simulink model "ggV_simu"  (R2019a)
settings: Solver=ode1  StartTime=0.0  StopTime=ggV.simu_stopTime  FixedStep=ggV.simu_stepSize  RelTol=1e-3
values from neighbouring files (symbols this model uses):
  init =     [course_data_0_1m.mat]
undefined symbols (not defined in the file or in its folder): ggV_v
settings Model: Creator=Frieder Uerlings  LastModifiedBy=Frieder Uerlings

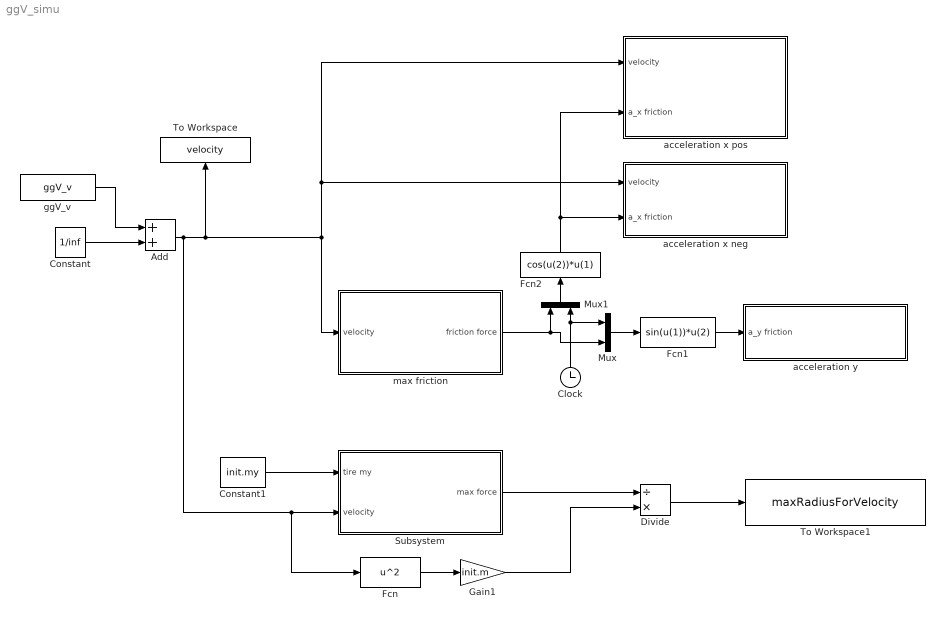
== system ggV_simu ==
  Add : Sum
  Clock : Clock
  Constant : Constant  Value=1/inf
  Constant1 : Constant  Value=init.my
  Divide : Product  Inputs=/*
  Fcn : Fcn  Expr=u^2
  Fcn1 : Fcn  Expr=sin(u(1))*u(2)
  Fcn2 : Fcn  Expr=cos(u(2))*u(1)
  Gain1 : Gain  Gain=init.m
  Mux : Mux  Inputs=2
  Mux1 : Mux  Inputs=2
  Subsystem : Subsystem
  To Workspace : ToWorkspace  VariableName=velocity  SampleTime=-1
  To Workspace1 : ToWorkspace  VariableName=maxRadiusForVelocity  SampleTime=-1
  acceleration x neg : Subsystem
  acceleration x pos : Subsystem
  acceleration y : Subsystem
  "ggV_v " : Constant  Value=ggV_v
  max friction : Subsystem
  wires:
  max friction/1(friction force) -> Mux1/1, Mux/2
  Fcn1/1 -> acceleration y/1(a_y friction)
  Fcn2/1 -> acceleration x pos/2(a_x friction), acceleration x neg/2(a_x friction)
  Add/1 -> Fcn/1, Subsystem/2(velocity), max friction/1(velocity), acceleration x neg/1(velocity), acceleration x pos/1(velocity), To Workspace/1
  Constant/1 -> Add/2
  "ggV_v "/1 -> Add/1
  Mux/1 -> Fcn1/1
  Mux1/1 -> Fcn2/1
  Clock/1 -> Mux/1, Mux1/2
  Divide/1 -> To Workspace1/1
  Gain1/1 -> Divide/2
  Constant1/1 -> Subsystem/1(tire my)
  Subsystem/1(max force) -> Divide/1
  Fcn/1 -> Gain1/1

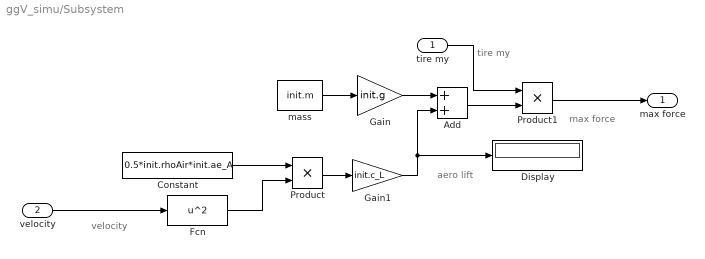
== system ggV_simu/Subsystem ==
  note: max force
  note: aero lift
  note: tire my
  note: velocity
  tire my : Inport
  velocity : Inport  Port=2
  Add : Sum
  Constant : Constant  Value=0.5*init.rhoAir*init.ae_A
  Display : Display
  Fcn : Fcn  Expr=u^2
  Gain : Gain  Gain=init.g
  Gain1 : Gain  Gain=init.c_L
  Product : Product
  Product1 : Product
  "mass " : Constant  Value=init.m
  max force : Outport
  wires:
  Constant/1 -> Product/1
  Add/1 -> Product1/2
  "mass "/1 -> Gain/1
  Fcn/1 -> Product/2
  Product1/1 -> max force/1
  Gain/1 -> Add/1
  Product/1 -> Gain1/1
  tire my/1 -> Product1/1
  velocity/1 -> Fcn/1
  Gain1/1 -> Add/2, Display/1

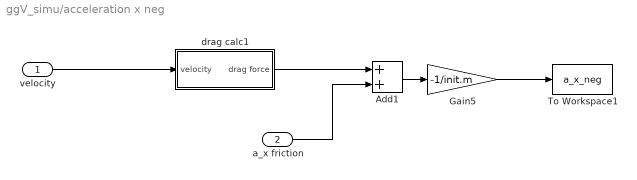
== system ggV_simu/acceleration x neg ==
  velocity : Inport
  a_x friction : Inport  Port=2
  Add1 : Sum
  Gain5 : Gain  Gain=-1/init.m
  To Workspace1 : ToWorkspace  VariableName=a_x_neg  SampleTime=-1
  drag calc1 : Subsystem
  wires:
  Add1/1 -> Gain5/1
  Gain5/1 -> To Workspace1/1
  velocity/1 -> drag calc1/1(velocity)
  a_x friction/1 -> Add1/2
  drag calc1/1("drag force ") -> Add1/1

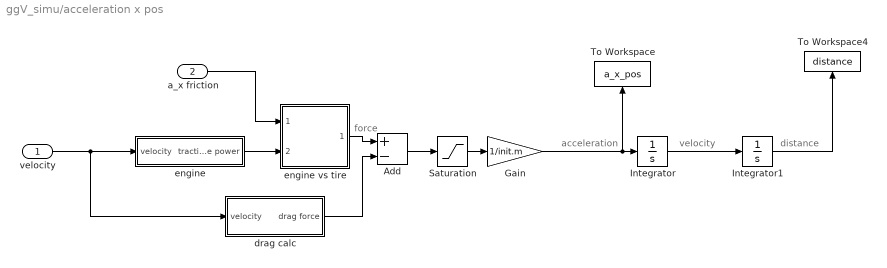
== system ggV_simu/acceleration x pos ==
  note: velocity
  note: force
  note: distance
  note: acceleration
  velocity : Inport
  a_x friction : Inport  Port=2
  Add : Sum  Inputs=+-
  Gain : Gain  Gain=1/init.m
  Integrator : Integrator
  Integrator1 : Integrator
  Saturation : Saturate  UpperLimit=inf  LowerLimit=0
  To Workspace : ToWorkspace  VariableName=a_x_pos  SampleTime=-1
  To Workspace4 : ToWorkspace  VariableName=distance  SampleTime=-1
  drag calc : Subsystem
  engine : Subsystem
  engine vs tire : Subsystem
  wires:
  engine vs tire/1(acc force) -> Add/1
  Gain/1 -> To Workspace/1, Integrator/1
  Integrator/1 -> Integrator1/1
  Add/1 -> Saturation/1
  Integrator1/1 -> To Workspace4/1
  drag calc/1("drag force ") -> Add/2
  engine/1(tractive power) -> engine vs tire/2(tractive power)
  a_x friction/1 -> engine vs tire/1("a_x friction ")
  velocity/1 -> drag calc/1(velocity), engine/1(velocity)
  Saturation/1 -> Gain/1

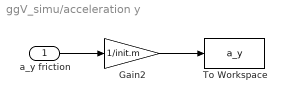
== system ggV_simu/acceleration y ==
  a_y friction : Inport
  Gain2 : Gain  Gain=1/init.m
  To Workspace : ToWorkspace  VariableName=a_y  SampleTime=-1
  wires:
  Gain2/1 -> To Workspace/1
  a_y friction/1 -> Gain2/1

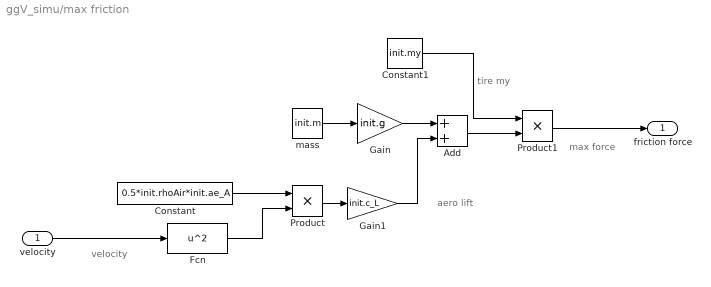
== system ggV_simu/max friction ==
  note: max force
  note: aero lift
  note: tire my
  note: velocity
  velocity : Inport
  Add : Sum
  Constant : Constant  Value=0.5*init.rhoAir*init.ae_A
  Constant1 : Constant  Value=init.my
  Fcn : Fcn  Expr=u^2
  Gain : Gain  Gain=init.g
  Gain1 : Gain  Gain=init.c_L
  Product : Product
  Product1 : Product
  "mass " : Constant  Value=init.m
  friction force : Outport
  wires:
  Constant/1 -> Product/1
  Add/1 -> Product1/2
  "mass "/1 -> Gain/1
  Fcn/1 -> Product/2
  Product1/1 -> friction force/1
  Gain/1 -> Add/1
  Product/1 -> Gain1/1
  Constant1/1 -> Product1/1
  velocity/1 -> Fcn/1
  Gain1/1 -> Add/2

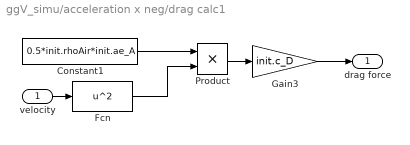
== system ggV_simu/acceleration x neg/drag calc1 ==
  velocity : Inport
  Constant1 : Constant  Value=0.5*init.rhoAir*init.ae_A
  Fcn : Fcn  Expr=u^2
  Gain3 : Gain  Gain=init.c_D
  Product : Product
  "drag force " : Outport
  wires:
  Gain3/1 -> "drag force "/1
  Product/1 -> Gain3/1
  Fcn/1 -> Product/2
  velocity/1 -> Fcn/1
  Constant1/1 -> Product/1

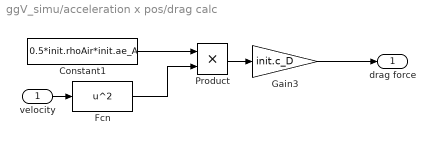
== system ggV_simu/acceleration x pos/drag calc ==
  velocity : Inport
  Constant1 : Constant  Value=0.5*init.rhoAir*init.ae_A
  Fcn : Fcn  Expr=u^2
  Gain3 : Gain  Gain=init.c_D
  Product : Product
  "drag force " : Outport
  wires:
  Constant1/1 -> Product/1
  velocity/1 -> Fcn/1
  Fcn/1 -> Product/2
  Product/1 -> Gain3/1
  Gain3/1 -> "drag force "/1

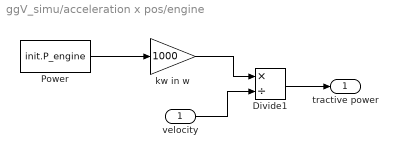
== system ggV_simu/acceleration x pos/engine ==
  velocity : Inport
  Divide1 : Product  Inputs=*/
  "Power " : Constant  Value=init.P_engine
  "kw in w " : Gain  Gain=1000
  tractive power : Outport
  wires:
  "Power "/1 -> "kw in w "/1
  "kw in w "/1 -> Divide1/1
  Divide1/1 -> tractive power/1
  velocity/1 -> Divide1/2

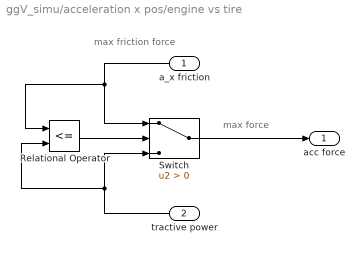
== system ggV_simu/acceleration x pos/engine vs tire ==
  note: max force
  note: max friction force
  "a_x friction " : Inport
  tractive power : Inport  Port=2
  Relational Operator : RelationalOperator  Operator=<=  OutDataTypeStr=boolean  RndMeth=Simplest
  Switch : Switch  Criteria=u2 > Threshold
  acc force : Outport
  wires:
  tractive power/1 -> Relational Operator/2, Switch/3
  "a_x friction "/1 -> Relational Operator/1, Switch/1
  Switch/1 -> acc force/1
  Relational Operator/1 -> Switch/2
